simulink model "symulacja_rs"  (R2016a)
settings: Solver=ode3  SolverMode=SingleTasking  StartTime=0.0  StopTime=10.0  RelTol=1e-3
values from neighbouring files (symbols this model uses):
  A = [-(Fzm*dz*cw+kw)/(mm*cwym) kw/(mm*cwym) 0 0 0 0 0 (Fzm*dz*cw)/(mm*cwym) ... (first row only)    [run_rs.m]
  B = [0 0 0 0 0 0 0 0]'    [run_rs.m]
  C = [1 0 0 0 0 0 0 0 ... (first row only)    [run_rs.m]
  D = [0 0 0 0 0 0]'    [run_rs.m]
  init = [Tpm_in Tzco_in Tpco1_in Tr1_in Tpco2_in Tr2_in To Tzm]    [run_rs.m]
settings Model: Creator=Piotr  LastModifiedBy=Piotr
settings DataIOCC: LimitDataPoints=on  SaveFormat=Array  SignalLoggingSaveFormat=ModelDataLogs
settings OptimizationCC: BlockReduction=off  BooleanDataType=off  ExpressionDepthLimit=2147483647
settings DebuggingCC: SaveWithParameterizedLinksMsg=none  UnderspecifiedInitializationDetection=Classic  MergeDetectMultiDrivingBlocksExec=none  SignalResolutionControl=TryResolveAllWithWarning  MultiTaskDSMMsg=warning  MultiTaskCondExecSysMsg=none  FcnCallInpInsideContextMsg=EnableAllAsWarning  StateNameClashWarn=warning
settings HardwareCC: ProdBitPerPointer=32  ProdLargestAtomicFloat=None  ProdIntDivRoundTo=Undefined  ProdEndianess=Unspecified  ProdWordSize=32  ProdHWDeviceType=32-bit Generic  TargetUnknown=on
settings ModelReferenceCC: PropagateSignalLabelsOutOfModel=off
settings ConfigComp: CovModelRefEnable=Off

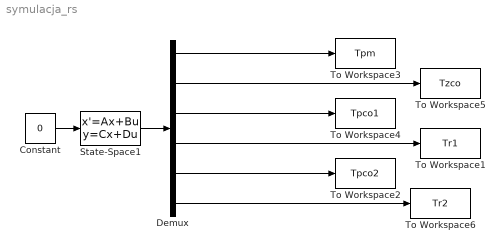
== system symulacja_rs ==
  Constant : Constant  Value=0
  Demux : Demux  Outputs=6
  State-Space1 : StateSpace  A=A  B=B  C=C  D=D  X0=init
  To Workspace1 : ToWorkspace  VariableName=Tr1  SampleTime=-1
  To Workspace2 : ToWorkspace  VariableName=Tpco2  SampleTime=-1
  To Workspace3 : ToWorkspace  VariableName=Tpm  SampleTime=-1
  To Workspace4 : ToWorkspace  VariableName=Tpco1  SampleTime=-1
  To Workspace5 : ToWorkspace  VariableName=Tzco  SampleTime=-1
  To Workspace6 : ToWorkspace  VariableName=Tr2  SampleTime=-1
  wires:
  Demux/3 -> To Workspace4/1
  State-Space1/1 -> Demux/1
  Constant/1 -> State-Space1/1
  Demux/2 -> To Workspace5/1
  Demux/1 -> To Workspace3/1
  Demux/4 -> To Workspace1/1
  Demux/5 -> To Workspace2/1
  Demux/6 -> To Workspace6/1
